simulink model "Wind_Turbine_test"  (R2023b)
settings: Solver=VariableStepAuto  StartTime=0.0  StopTime=1  RelTol=1e-3
model workspace (MAT data in the model file):
  Compensation_Ki = 30
  Compensation_Kp = 3
  DC_Ki = 400
  DC_Kp = 8
  F = 0.01
  Flux_min = 0.5
  Grid_Freq_PWM = 2700
  Grid_Ireg_Ki = 5
  Grid_Ireg_Kp = 0.83
  Grid_Ireg_lim = 1.1
  Grid_Modindex_Upper = 1.1
  Grid_conv_Imax = 0.8
  H = 0.685
  Idref_max = 0.9
  Iqref_Tc = 0.3
  Ki_Var = 0.05
  Ki_Vreg = 20
  Ksh = 1.1
  L_pu = 0.3
  Llr = 0.16
  Lls = 0.18
  Lm = 2.9
  P_mech = 1080000
  Pitch_Ki = 0
  Pitch_Kp = 150
  Pitch_Max = 27
  Pitch_Tc = 0.01
  Pitch_rate = 10
  Q_Filt = 50
  R_pu = 0.003
  Rotor_Freq_PWM = 1620
  Rotor_Ireg_Ki = 8
  Rotor_Ireg_Kp = 0.6
  Rotor_Ireg_lim = 0.1
  Rotor_Modindex_Upper = 2
  Rr = 0.016
  Rs = 0.023
  T_set = 0.0001
  Tp = 5e-05
  Ts = 5e-06
  Var_C_Filt = 720000
  Var_reg_max = 1.1
  Var_reg_min = 0.9
  WT_Coeff = [0.645 116 0.4 5 21 0.00912 0.08 0.035]
  WT_H = 4.32
  WT_IGBTRon = 5.931
  WT_Param = [91.204 10143]
  Wind_Freq_Filt = 10000
  Wind_Freq_nom = 60
  Wind_P_nom = 1200000
  Wind_Rotor_V_nom = 1950
  Wind_V_nom = 500
  Zeta_Filt = 0.707106781187
  init = [-0.2 0 0 0 0 0 0 0]
  p = 3
  torque0 = 0.83
  v_Ki = 0.1
  v_Kp = 3.6
  v_Max = 1.2
  v_Min = 0.7
  v_T = 5
  vreg_max = 1
  wind_VDC_nom = 1150
  wt0 = 1.2
undefined symbols (not defined in the file): D1, D11, Delta, DiscIntNeverNeededParam, P, Q
libraries: powerlib_extras x144, simulink_extras x24, spsThreePhaseVIMeasurementLib x13, spsThreePhaseTransformerTwoWindingsLib x11, spsSeriesRLCBranchLib x9, spsPWMGenerator2LevelLib x8, spsUniversalBridgeLib x8, spsThreePhaseSeriesRLCLoadLib x6, spsThreePhasePISectionLineLib x5, spsGroundLib x5, spsLoadFlowBusLib x4, spsAsynchronousMachinepuUnitsLib x4
(part 4 of 9)

== system Wind_Turbine_test/Wind Farm/Wind Turbine 1/Wind Turbine & Generator 1/Shaft ==
  Speed : Inport
  Discrete-Time Integrator1 : DiscreteIntegrator  InitialCondition=torque0/Ksh  SampleTime=Ts  ICPrevOutput=DiscIntNeverNeededParam  ICPrevScaledInput=DiscIntNeverNeededParam
  Mutual damping : Gain  Gain=1.5  SaturateOnIntegerOverflow=on  OutDataTypeStr=Inherit: Same as input  ParamDataTypeStr=Inherit: Same as input
  Stiffness : Gain  Gain=Ksh  SaturateOnIntegerOverflow=on  OutDataTypeStr=Inherit: Same as input  ParamDataTypeStr=Inherit: Same as input
  Sum2 : Sum  InputSameDT=on  SaturateOnIntegerOverflow=on  OutDataTypeStr=Inherit: Same as first input
  wbase : Gain  Gain=125.7  SaturateOnIntegerOverflow=on  OutDataTypeStr=Inherit: Same as input  ParamDataTypeStr=Inherit: Same as input
  T_shaft (pu) : Outport  VectorParamsAs1DForOutWhenUnconnected=off
  wires:
  Mutual damping/1 -> Sum2/2
  Stiffness/1 -> Sum2/1
  Sum2/1 -> T_shaft (pu)/1
  Speed/1 -> Mutual damping/1, wbase/1
  Discrete-Time Integrator1/1 -> Stiffness/1
  wbase/1 -> Discrete-Time Integrator1/1

== system Wind_Turbine_test/Wind Farm/Wind Turbine 1/Wind Turbine & Generator 1/Turbine ==
  T_wt (pu) : Inport
  T_shaft (pu) : Inport  Port=2
  Generator speed (pu) : Inport  Port=3
  1_2H_WT : Gain  Gain=1/(2*WT_H)  SaturateOnIntegerOverflow=on  OutDataTypeStr=Inherit: Same as input  ParamDataTypeStr=Inherit: Same as input
  Discrete-Time Integrator : DiscreteIntegrator  InitialCondition=wt0  SampleTime=Ts  ICPrevOutput=DiscIntNeverNeededParam  ICPrevScaledInput=DiscIntNeverNeededParam
  Sum : Sum  Inputs=+-  InputSameDT=on  SaturateOnIntegerOverflow=on  OutDataTypeStr=Inherit: Same as first input
  Sum1 : Sum  Inputs=+-  InputSameDT=on  SaturateOnIntegerOverflow=on  OutDataTypeStr=Inherit: Same as first input
  Turbine speed : Outport
  W_wt (pu) : Outport  Port=2  VectorParamsAs1DForOutWhenUnconnected=off
  wires:
  Sum1/1 -> Turbine speed/1
  Sum/1 -> 1_2H_WT/1
  Discrete-Time Integrator/1 -> W_wt (pu)/1, Sum1/1
  1_2H_WT/1 -> Discrete-Time Integrator/1
  T_wt (pu)/1 -> Sum/1
  T_shaft (pu)/1 -> Sum/2
  Generator speed (pu)/1 -> Sum1/2

== system Wind_Turbine_test/Wind Farm/Wind Turbine 1/Wind Turbine & Generator 1/Wind Turbine  ==
  Generator speed (pu)1 : Inport
  Pitch angle (deg) : Inport  Port=2
  Wind speed (m/s) : Inport  Port=3
  ->pu : Gain  Gain=1/Pmech_Out
  Avoid div. by zero : Saturate  UpperLimit=inf  LowerLimit=eps
  "Avoid div. by zero " : Saturate  UpperLimit=inf  LowerLimit=eps
  Fcn1 : Fcn  Expr=WT_Param(1)*u[2]/u[1]
  Fcn2 : Fcn  Expr=WT_Coeff8(1)*(WT_Coeff8(6)*u[1] + (-WT_Coeff8(4) - WT_Coeff8(3)*(2.5 + u[2]) + WT_Coeff8(2)*(1/(u[1] + WT_Coeff8(7)*(2.5 + u[2])) -WT_Coeff8(8)/(1 + (2.5 + u[2])^3)))/exp(WT_Coeff8(5)*(1/(u[1] + WT_Coeff8(7)*(2.5 + u[2])) - WT_Coeff8(8)/(1 + (2.5 + u[2])^3))))
  "K2*Cp*wind^3 " : Fcn  Expr=WT_Param(2)*u[1]^3*u[2]
  Mux : Mux  Inputs=2
  Mux1 : Mux  Inputs=2
  Mux2 : Mux  Inputs=2
  Product2 : Product  Inputs=*/  InputSameDT=on  SaturateOnIntegerOverflow=on  OutDataTypeStr=Inherit: Same as first input
  Tt (pu) : Outport  VectorParamsAs1DForOutWhenUnconnected=off
  wires:
  Generator speed (pu)1/1 -> "Avoid div. by zero "/1
  Mux1/1 -> Fcn2/1
  ->pu/1 -> Product2/1  "power_pu"
  Avoid div. by zero/1 -> Mux/1, Mux2/1
  "Avoid div. by zero "/1 -> Product2/2, Mux/2
  "K2*Cp*wind^3 "/1 -> ->pu/1
  Mux2/1 -> "K2*Cp*wind^3 "/1
  Fcn1/1 -> Mux1/1  "lambda"
  Mux/1 -> Fcn1/1
  Pitch angle (deg)/1 -> Mux1/2
  Wind speed (m/s)/1 -> Avoid div. by zero/1
  Product2/1 -> Tt (pu)/1
  Fcn2/1 -> Mux2/2  "Cp"

== system Wind_Turbine_test/Wind Farm/Wind Turbine 2/Wind Turbine & Generator 1/Shaft ==
  Speed : Inport
  Discrete-Time Integrator1 : DiscreteIntegrator  InitialCondition=torque0/Ksh  SampleTime=Ts  ICPrevOutput=DiscIntNeverNeededParam  ICPrevScaledInput=DiscIntNeverNeededParam
  Mutual damping : Gain  Gain=1.5  SaturateOnIntegerOverflow=on  OutDataTypeStr=Inherit: Same as input  ParamDataTypeStr=Inherit: Same as input
  Stiffness : Gain  Gain=Ksh  SaturateOnIntegerOverflow=on  OutDataTypeStr=Inherit: Same as input  ParamDataTypeStr=Inherit: Same as input
  Sum2 : Sum  InputSameDT=on  SaturateOnIntegerOverflow=on  OutDataTypeStr=Inherit: Same as first input
  wbase : Gain  Gain=125.7  SaturateOnIntegerOverflow=on  OutDataTypeStr=Inherit: Same as input  ParamDataTypeStr=Inherit: Same as input
  T_shaft (pu) : Outport  VectorParamsAs1DForOutWhenUnconnected=off
  wires:
  Mutual damping/1 -> Sum2/2
  Stiffness/1 -> Sum2/1
  Sum2/1 -> T_shaft (pu)/1
  Speed/1 -> Mutual damping/1, wbase/1
  Discrete-Time Integrator1/1 -> Stiffness/1
  wbase/1 -> Discrete-Time Integrator1/1

== system Wind_Turbine_test/Wind Farm/Wind Turbine 2/Wind Turbine & Generator 1/Turbine ==
  T_wt (pu) : Inport
  T_shaft (pu) : Inport  Port=2
  Generator speed (pu) : Inport  Port=3
  1_2H_WT : Gain  Gain=1/(2*WT_H)  SaturateOnIntegerOverflow=on  OutDataTypeStr=Inherit: Same as input  ParamDataTypeStr=Inherit: Same as input
  Discrete-Time Integrator : DiscreteIntegrator  InitialCondition=wt0  SampleTime=Ts  ICPrevOutput=DiscIntNeverNeededParam  ICPrevScaledInput=DiscIntNeverNeededParam
  Sum : Sum  Inputs=+-  InputSameDT=on  SaturateOnIntegerOverflow=on  OutDataTypeStr=Inherit: Same as first input
  Sum1 : Sum  Inputs=+-  InputSameDT=on  SaturateOnIntegerOverflow=on  OutDataTypeStr=Inherit: Same as first input
  Turbine speed : Outport
  W_wt (pu) : Outport  Port=2  VectorParamsAs1DForOutWhenUnconnected=off
  wires:
  Sum1/1 -> Turbine speed/1
  Sum/1 -> 1_2H_WT/1
  Discrete-Time Integrator/1 -> W_wt (pu)/1, Sum1/1
  1_2H_WT/1 -> Discrete-Time Integrator/1
  T_wt (pu)/1 -> Sum/1
  T_shaft (pu)/1 -> Sum/2
  Generator speed (pu)/1 -> Sum1/2

== system Wind_Turbine_test/Wind Farm/Wind Turbine 2/Wind Turbine & Generator 1/Wind Turbine  ==
  Generator speed (pu)1 : Inport
  Pitch angle (deg) : Inport  Port=2
  Wind speed (m/s) : Inport  Port=3
  ->pu : Gain  Gain=1/Pmech_Out
  Avoid div. by zero : Saturate  UpperLimit=inf  LowerLimit=eps
  "Avoid div. by zero " : Saturate  UpperLimit=inf  LowerLimit=eps
  Fcn1 : Fcn  Expr=WT_Param(1)*u[2]/u[1]
  Fcn2 : Fcn  Expr=WT_Coeff8(1)*(WT_Coeff8(6)*u[1] + (-WT_Coeff8(4) - WT_Coeff8(3)*(2.5 + u[2]) + WT_Coeff8(2)*(1/(u[1] + WT_Coeff8(7)*(2.5 + u[2])) -WT_Coeff8(8)/(1 + (2.5 + u[2])^3)))/exp(WT_Coeff8(5)*(1/(u[1] + WT_Coeff8(7)*(2.5 + u[2])) - WT_Coeff8(8)/(1 + (2.5 + u[2])^3))))
  "K2*Cp*wind^3 " : Fcn  Expr=WT_Param(2)*u[1]^3*u[2]
  Mux : Mux  Inputs=2
  Mux1 : Mux  Inputs=2
  Mux2 : Mux  Inputs=2
  Product2 : Product  Inputs=*/  InputSameDT=on  SaturateOnIntegerOverflow=on  OutDataTypeStr=Inherit: Same as first input
  Tt (pu) : Outport  VectorParamsAs1DForOutWhenUnconnected=off
  wires:
  Generator speed (pu)1/1 -> "Avoid div. by zero "/1
  Mux1/1 -> Fcn2/1
  ->pu/1 -> Product2/1  "power_pu"
  Avoid div. by zero/1 -> Mux/1, Mux2/1
  "Avoid div. by zero "/1 -> Product2/2, Mux/2
  "K2*Cp*wind^3 "/1 -> ->pu/1
  Mux2/1 -> "K2*Cp*wind^3 "/1
  Fcn1/1 -> Mux1/1  "lambda"
  Mux/1 -> Fcn1/1
  Pitch angle (deg)/1 -> Mux1/2
  Wind speed (m/s)/1 -> Avoid div. by zero/1
  Product2/1 -> Tt (pu)/1
  Fcn2/1 -> Mux2/2  "Cp"

== system Wind_Turbine_test/Wind Farm/Wind Turbine 3/Wind Turbine & Generator 1/Shaft ==
  Speed : Inport
  Discrete-Time Integrator1 : DiscreteIntegrator  InitialCondition=torque0/Ksh  SampleTime=Ts  ICPrevOutput=DiscIntNeverNeededParam  ICPrevScaledInput=DiscIntNeverNeededParam
  Mutual damping : Gain  Gain=1.5  SaturateOnIntegerOverflow=on  OutDataTypeStr=Inherit: Same as input  ParamDataTypeStr=Inherit: Same as input
  Stiffness : Gain  Gain=Ksh  SaturateOnIntegerOverflow=on  OutDataTypeStr=Inherit: Same as input  ParamDataTypeStr=Inherit: Same as input
  Sum2 : Sum  InputSameDT=on  SaturateOnIntegerOverflow=on  OutDataTypeStr=Inherit: Same as first input
  wbase : Gain  Gain=125.7  SaturateOnIntegerOverflow=on  OutDataTypeStr=Inherit: Same as input  ParamDataTypeStr=Inherit: Same as input
  T_shaft (pu) : Outport  VectorParamsAs1DForOutWhenUnconnected=off
  wires:
  Mutual damping/1 -> Sum2/2
  Stiffness/1 -> Sum2/1
  Sum2/1 -> T_shaft (pu)/1
  Speed/1 -> Mutual damping/1, wbase/1
  Discrete-Time Integrator1/1 -> Stiffness/1
  wbase/1 -> Discrete-Time Integrator1/1

== system Wind_Turbine_test/Wind Farm/Wind Turbine 3/Wind Turbine & Generator 1/Turbine ==
  T_wt (pu) : Inport
  T_shaft (pu) : Inport  Port=2
  Generator speed (pu) : Inport  Port=3
  1_2H_WT : Gain  Gain=1/(2*WT_H)  SaturateOnIntegerOverflow=on  OutDataTypeStr=Inherit: Same as input  ParamDataTypeStr=Inherit: Same as input
  Discrete-Time Integrator : DiscreteIntegrator  InitialCondition=wt0  SampleTime=Ts  ICPrevOutput=DiscIntNeverNeededParam  ICPrevScaledInput=DiscIntNeverNeededParam
  Sum : Sum  Inputs=+-  InputSameDT=on  SaturateOnIntegerOverflow=on  OutDataTypeStr=Inherit: Same as first input
  Sum1 : Sum  Inputs=+-  InputSameDT=on  SaturateOnIntegerOverflow=on  OutDataTypeStr=Inherit: Same as first input
  Turbine speed : Outport
  W_wt (pu) : Outport  Port=2  VectorParamsAs1DForOutWhenUnconnected=off
  wires:
  Sum1/1 -> Turbine speed/1
  Sum/1 -> 1_2H_WT/1
  Discrete-Time Integrator/1 -> W_wt (pu)/1, Sum1/1
  1_2H_WT/1 -> Discrete-Time Integrator/1
  T_wt (pu)/1 -> Sum/1
  T_shaft (pu)/1 -> Sum/2
  Generator speed (pu)/1 -> Sum1/2

== system Wind_Turbine_test/Wind Farm/Wind Turbine 3/Wind Turbine & Generator 1/Wind Turbine  ==
  Generator speed (pu)1 : Inport
  Pitch angle (deg) : Inport  Port=2
  Wind speed (m/s) : Inport  Port=3
  ->pu : Gain  Gain=1/Pmech_Out
  Avoid div. by zero : Saturate  UpperLimit=inf  LowerLimit=eps
  "Avoid div. by zero " : Saturate  UpperLimit=inf  LowerLimit=eps
  Fcn1 : Fcn  Expr=WT_Param(1)*u[2]/u[1]
  Fcn2 : Fcn  Expr=WT_Coeff8(1)*(WT_Coeff8(6)*u[1] + (-WT_Coeff8(4) - WT_Coeff8(3)*(2.5 + u[2]) + WT_Coeff8(2)*(1/(u[1] + WT_Coeff8(7)*(2.5 + u[2])) -WT_Coeff8(8)/(1 + (2.5 + u[2])^3)))/exp(WT_Coeff8(5)*(1/(u[1] + WT_Coeff8(7)*(2.5 + u[2])) - WT_Coeff8(8)/(1 + (2.5 + u[2])^3))))
  "K2*Cp*wind^3 " : Fcn  Expr=WT_Param(2)*u[1]^3*u[2]
  Mux : Mux  Inputs=2
  Mux1 : Mux  Inputs=2
  Mux2 : Mux  Inputs=2
  Product2 : Product  Inputs=*/  InputSameDT=on  SaturateOnIntegerOverflow=on  OutDataTypeStr=Inherit: Same as first input
  Tt (pu) : Outport  VectorParamsAs1DForOutWhenUnconnected=off
  wires:
  Generator speed (pu)1/1 -> "Avoid div. by zero "/1
  Mux1/1 -> Fcn2/1
  ->pu/1 -> Product2/1  "power_pu"
  Avoid div. by zero/1 -> Mux/1, Mux2/1
  "Avoid div. by zero "/1 -> Product2/2, Mux/2
  "K2*Cp*wind^3 "/1 -> ->pu/1
  Mux2/1 -> "K2*Cp*wind^3 "/1
  Fcn1/1 -> Mux1/1  "lambda"
  Mux/1 -> Fcn1/1
  Pitch angle (deg)/1 -> Mux1/2
  Wind speed (m/s)/1 -> Avoid div. by zero/1
  Product2/1 -> Tt (pu)/1
  Fcn2/1 -> Mux2/2  "Cp"

== system Wind_Turbine_test/Wind Farm/Wind Turbine 4/Wind Turbine & Generator 1/Shaft ==
  Speed : Inport
  Discrete-Time Integrator1 : DiscreteIntegrator  InitialCondition=torque0/Ksh  SampleTime=Ts  ICPrevOutput=DiscIntNeverNeededParam  ICPrevScaledInput=DiscIntNeverNeededParam
  Mutual damping : Gain  Gain=1.5  SaturateOnIntegerOverflow=on  OutDataTypeStr=Inherit: Same as input  ParamDataTypeStr=Inherit: Same as input
  Stiffness : Gain  Gain=Ksh  SaturateOnIntegerOverflow=on  OutDataTypeStr=Inherit: Same as input  ParamDataTypeStr=Inherit: Same as input
  Sum2 : Sum  InputSameDT=on  SaturateOnIntegerOverflow=on  OutDataTypeStr=Inherit: Same as first input
  wbase : Gain  Gain=125.7  SaturateOnIntegerOverflow=on  OutDataTypeStr=Inherit: Same as input  ParamDataTypeStr=Inherit: Same as input
  T_shaft (pu) : Outport  VectorParamsAs1DForOutWhenUnconnected=off
  wires:
  Mutual damping/1 -> Sum2/2
  Stiffness/1 -> Sum2/1
  Sum2/1 -> T_shaft (pu)/1
  Speed/1 -> Mutual damping/1, wbase/1
  Discrete-Time Integrator1/1 -> Stiffness/1
  wbase/1 -> Discrete-Time Integrator1/1

== system Wind_Turbine_test/Wind Farm/Wind Turbine 4/Wind Turbine & Generator 1/Turbine ==
  T_wt (pu) : Inport
  T_shaft (pu) : Inport  Port=2
  Generator speed (pu) : Inport  Port=3
  1_2H_WT : Gain  Gain=1/(2*WT_H)  SaturateOnIntegerOverflow=on  OutDataTypeStr=Inherit: Same as input  ParamDataTypeStr=Inherit: Same as input
  Discrete-Time Integrator : DiscreteIntegrator  InitialCondition=wt0  SampleTime=Ts  ICPrevOutput=DiscIntNeverNeededParam  ICPrevScaledInput=DiscIntNeverNeededParam
  Sum : Sum  Inputs=+-  InputSameDT=on  SaturateOnIntegerOverflow=on  OutDataTypeStr=Inherit: Same as first input
  Sum1 : Sum  Inputs=+-  InputSameDT=on  SaturateOnIntegerOverflow=on  OutDataTypeStr=Inherit: Same as first input
  Turbine speed : Outport
  W_wt (pu) : Outport  Port=2  VectorParamsAs1DForOutWhenUnconnected=off
  wires:
  Sum1/1 -> Turbine speed/1
  Sum/1 -> 1_2H_WT/1
  Discrete-Time Integrator/1 -> W_wt (pu)/1, Sum1/1
  1_2H_WT/1 -> Discrete-Time Integrator/1
  T_wt (pu)/1 -> Sum/1
  T_shaft (pu)/1 -> Sum/2
  Generator speed (pu)/1 -> Sum1/2

== system Wind_Turbine_test/Wind Farm/Wind Turbine 4/Wind Turbine & Generator 1/Wind Turbine  ==
  Generator speed (pu)1 : Inport
  Pitch angle (deg) : Inport  Port=2
  Wind speed (m/s) : Inport  Port=3
  ->pu : Gain  Gain=1/Pmech_Out
  Avoid div. by zero : Saturate  UpperLimit=inf  LowerLimit=eps
  "Avoid div. by zero " : Saturate  UpperLimit=inf  LowerLimit=eps
  Fcn1 : Fcn  Expr=WT_Param(1)*u[2]/u[1]
  Fcn2 : Fcn  Expr=WT_Coeff8(1)*(WT_Coeff8(6)*u[1] + (-WT_Coeff8(4) - WT_Coeff8(3)*(2.5 + u[2]) + WT_Coeff8(2)*(1/(u[1] + WT_Coeff8(7)*(2.5 + u[2])) -WT_Coeff8(8)/(1 + (2.5 + u[2])^3)))/exp(WT_Coeff8(5)*(1/(u[1] + WT_Coeff8(7)*(2.5 + u[2])) - WT_Coeff8(8)/(1 + (2.5 + u[2])^3))))
  "K2*Cp*wind^3 " : Fcn  Expr=WT_Param(2)*u[1]^3*u[2]
  Mux : Mux  Inputs=2
  Mux1 : Mux  Inputs=2
  Mux2 : Mux  Inputs=2
  Product2 : Product  Inputs=*/  InputSameDT=on  SaturateOnIntegerOverflow=on  OutDataTypeStr=Inherit: Same as first input
  Tt (pu) : Outport  VectorParamsAs1DForOutWhenUnconnected=off
  wires:
  Generator speed (pu)1/1 -> "Avoid div. by zero "/1
  Mux1/1 -> Fcn2/1
  ->pu/1 -> Product2/1  "power_pu"
  Avoid div. by zero/1 -> Mux/1, Mux2/1
  "Avoid div. by zero "/1 -> Product2/2, Mux/2
  "K2*Cp*wind^3 "/1 -> ->pu/1
  Mux2/1 -> "K2*Cp*wind^3 "/1
  Fcn1/1 -> Mux1/1  "lambda"
  Mux/1 -> Fcn1/1
  Pitch angle (deg)/1 -> Mux1/2
  Wind speed (m/s)/1 -> Avoid div. by zero/1
  Product2/1 -> Tt (pu)/1
  Fcn2/1 -> Mux2/2  "Cp"

== system Wind_Turbine_test/Wind Farm/Control System/Control System 1/Grid-side Control System/Current Regulator ==
  Stator_Vdq : Inport
  In2 : Inport  Port=2
  Grid_conv_Idq : Inport  Port=3
  w : Inport  Port=4
  Constant1 : Constant  Value=L_pu
  Constant2 : Constant  Value=L_pu
  Constant3 : Constant  Value=R_pu
  Constant4 : Constant  Value=R_pu
  Demux{,1..3} (4 alike) : Demux  Outputs=2
      settings: DisplayOption=none
  Discrete PI Controller1 : powerlib_extras/Discrete  Control Blocks/Discrete PI Controller  Kp=Grid_Ireg_Kp  Ki=Grid_Ireg_Ki  Par_Limits=[1.0 -1.0] *Grid_Ireg_lim  Init=0  Ts=Ts
  Mux2 : Mux  Inputs=2
  Product : Product  Inputs=3  InputSameDT=on  SaturateOnIntegerOverflow=on  OutDataTypeStr=Inherit: Same as first input
  Product1 : Product  Inputs=3  InputSameDT=on  SaturateOnIntegerOverflow=on  OutDataTypeStr=Inherit: Same as first input
  Product2 : Product  InputSameDT=on  SaturateOnIntegerOverflow=on  OutDataTypeStr=Inherit: Same as first input
  Product3 : Product  InputSameDT=on  SaturateOnIntegerOverflow=on  OutDataTypeStr=Inherit: Same as first input
  Sum1 : Sum  Inputs=+-  InputSameDT=on  SaturateOnIntegerOverflow=on  OutDataTypeStr=Inherit: Same as first input
  Sum2 : Sum  Inputs=-+|  InputSameDT=on  SaturateOnIntegerOverflow=on  OutDataTypeStr=Inherit: Same as first input
  Sum3 : Sum  Inputs=||++-  InputSameDT=on  SaturateOnIntegerOverflow=on  OutDataTypeStr=Inherit: Same as first input
  Sum4 : Sum  Inputs=|+-  InputSameDT=on  SaturateOnIntegerOverflow=on  OutDataTypeStr=Inherit: Same as first input
  Sum5 : Sum  Inputs=|--+  InputSameDT=on  SaturateOnIntegerOverflow=on  OutDataTypeStr=Inherit: Same as first input
  Sum6 : Sum  Inputs=|-+  InputSameDT=on  SaturateOnIntegerOverflow=on  OutDataTypeStr=Inherit: Same as first input
  Grid_conv_Vd : Outport
  Grid_conv_Vq : Outport  Port=2
  wires:
  Product1/1 -> Sum5/2
  Product2/1 -> Sum3/3
  Product3/1 -> Sum5/1
  [id_ref] -> Product2/2
  Sum1/1 -> Grid_conv_Vd/1  "Grid_conv_Vd"
  Demux1/2 -> [iq_ref], Sum2/2  "Iq_ref"
  Demux/1 -> Sum4/2  "Id"
  [w] -> Product/2
  Demux2/2 -> Sum5/3  "Vq"
  [iq_ref] -> Product/3
  Sum4/1 -> Mux2/1
  Constant4/1 -> Product3/2
  Stator_Vdq/1 -> Demux2/1
  Constant2/1 -> Product1/2
  Constant3/1 -> Product2/1
  Grid_conv_Idq/1 -> Demux/1
  Product/1 -> Sum3/2
  Discrete PI Controller1/1 -> Demux3/1
  Sum2/1 -> Mux2/2
  Sum6/1 -> Grid_conv_Vq/1  "Grid_conv_Vq"
  w/1 -> [w]
  [id_ref] -> Product1/1
  Sum5/1 -> Sum6/2
  [iq_ref] -> Product3/1
  Sum3/1 -> Sum1/1
  Mux2/1 -> Discrete PI Controller1/1
  Demux2/1 -> Sum3/1  "Vd"
  Demux1/1 -> Sum4/1, [id_ref]  "Id_ref"
  Demux3/1 -> Sum1/2  "vd'"
  Constant1/1 -> Product/1
  Demux/2 -> Sum2/1  "Iq"
  Demux3/2 -> Sum6/1  "vq'"
  [w] -> Product1/3
  In2/1 -> Demux1/1

== system Wind_Turbine_test/Wind Farm/Control System/Control System 1/Grid-side Control System/Grid Voltage Converter ==
  dq0 : Inport
  Theta_PLL : Inport  Port=2
  Mux5 : Mux  Inputs=2
  Trigonometric Function2 : Trigonometry
  Trigonometric Function3 : Trigonometry  Operator=cos
  dq0_to_abc Transformation : powerlib_extras/Measurements/dq0_to_abc Transformation
  Grid_conv_V : Outport  VectorParamsAs1DForOutWhenUnconnected=off
  wires:
  Trigonometric Function2/1 -> Mux5/1
  Mux5/1 -> dq0_to_abc Transformation/2
  Theta_PLL/1 -> Trigonometric Function2/1, Trigonometric Function3/1
  dq0_to_abc Transformation/1 -> Grid_conv_V/1
  dq0/1 -> dq0_to_abc Transformation/1
  Trigonometric Function3/1 -> Mux5/2

== system Wind_Turbine_test/Wind Farm/Control System/Control System 1/Grid-side Control System/Modulation ==
  x : Inport
  y : Inport  Port=2
  1 : Saturate  UpperLimit=Grid_Modindex_Upper  LowerLimit=0
  Avoid division by zero : Saturate  UpperLimit=inf  LowerLimit=1e-6
  Cartesian to Polar1 : simulink_extras/Transformations/Cartesian to Polar
  K : Constant  Value=Wind_V_nom*2*sqrt(2/3)
  Mux4 : Mux  Inputs=3
  Polar to Cartesian : simulink_extras/Transformations/Polar to Cartesian
  Product4 : Product  Inputs=**/  InputSameDT=on  SaturateOnIntegerOverflow=on  OutDataTypeStr=Inherit: Same as first input
  V0 : Constant  Value=0
  Vdq0 : Outport
  wires:
  K/1 -> Product4/2
  Polar to Cartesian/2 -> Mux4/2
  V0/1 -> Mux4/3
  y/1 -> Cartesian to Polar1/2
  [Vdc] -> Avoid division by zero/1
  Polar to Cartesian/1 -> Mux4/1
  Mux4/1 -> Vdq0/1  "Vdq0"
  Avoid division by zero/1 -> Product4/3
  1/1 -> Polar to Cartesian/1
  Cartesian to Polar1/2 -> Polar to Cartesian/2
  Product4/1 -> 1/1  "m"
  x/1 -> Cartesian to Polar1/1
  Cartesian to Polar1/1 -> Product4/1

== system Wind_Turbine_test/Wind Farm/Control System/Control System 1/Grid-side Control System/VDC Regulator ==
  Iq_ref : Inport
  Vdc : Inport  Port=2
  ->pu : Gain  Gain=1/wind_VDC_nom
  Discrete PI Controller : powerlib_extras/Discrete  Control Blocks/Discrete PI Controller  Kp=DC_Kp  Ki=DC_Ki  Par_Limits=[1 -1]*Grid_conv_Imax  Init=0  Ts=Ts
  Mux : Mux  Inputs=2
  Sum7 : Sum  Inputs=|+-  InputSameDT=on  SaturateOnIntegerOverflow=on  OutDataTypeStr=Inherit: Same as first input
  Vdc_ref (V) : Constant  Value=wind_VDC_nom
  Out1 : Outport
  wires:
  Vdc/1 -> [Vdc], Sum7/2
  Iq_ref/1 -> Mux/2
  Mux/1 -> Out1/1
  Discrete PI Controller/1 -> Mux/1  "Id_ref"
  ->pu/1 -> Discrete PI Controller/1
  Vdc_ref (V)/1 -> Sum7/1
  Sum7/1 -> ->pu/1

== system Wind_Turbine_test/Wind Farm/Control System/Control System 1/Measurement and abc-to-dq transformation / Improved Discrete 3-phase PLL ==
  note: Pierre Giroux, Gilbert Sybille, R. Gagnon
      | Power System Laboratory, IREQ
      | Hydro-Quebec
  note: New Discrete 3-phase PLL
  Vabc_pu : Inport  PortDimensions=3
  2nd-Order Filter : powerlib_extras/Discrete  Control Blocks/Discrete  2nd-Order Filter  FilterType=Lowpass  Fo=25  Zeta=0.707  Ts=Ts  Initialize=on  Vac_Init=[0 0 Finit]  Vdc_Init=Finit  PlotResponse=off  param1=[1 500 0.1]
  Constant1 : Constant  Value=2*pi*Finit
  Constant4 : Constant  Value=2*pi
  Discrete-Time Integrator : DiscreteIntegrator  SampleTime=Ts  ICPrevOutput=DiscIntNeverNeededParam  ICPrevScaledInput=DiscIntNeverNeededParam
  Discrete-Time Integrator1 : DiscreteIntegrator  gainval=1  SampleTime=Ts  LimitOutput=on  UpperSaturationLimit=2*pi*5  LowerSaturationLimit=-2*pi*5  ICPrevOutput=DiscIntNeverNeededParam  ICPrevScaledInput=DiscIntNeverNeededParam
  Gain10 : Gain  Gain=1/2/pi  SaturateOnIntegerOverflow=on  OutDataTypeStr=Inherit: Same as input  ParamDataTypeStr=Inherit: Same as input
  Kp1 : Gain  Gain=Kp2  SaturateOnIntegerOverflow=on  OutDataTypeStr=Inherit: Same as input  ParamDataTypeStr=Inherit: Same as input
  Kp2 : Gain  Gain=Ki2  SaturateOnIntegerOverflow=on  OutDataTypeStr=Inherit: Same as input  ParamDataTypeStr=Inherit: Same as input
  Kp3 : Gain  Gain=Ki1  SaturateOnIntegerOverflow=on  OutDataTypeStr=Inherit: Same as input  ParamDataTypeStr=Inherit: Same as input
  Kp4 : Gain  Gain=Kp1  SaturateOnIntegerOverflow=on  OutDataTypeStr=Inherit: Same as input  ParamDataTypeStr=Inherit: Same as input
  Math Function : Math  Operator=mod  SignedPower=on
  Mux2 : Mux  Inputs=2
  Rate Limiter : powerlib_extras/Discrete  Control Blocks/Discrete Rate Limiter  R=12  F=-12  Vinit=Finit  Ts=Ts
  Selector : Selector  InputPortWidth=3  IndexOptions=Index vector (dialog)  Indices=2  OutputSizes=1
  Sum : Sum  Inputs=+++
  Trigonometric Function : Trigonometry
  Trigonometric Function1 : Trigonometry  Operator=atan
  Trigonometric Function2 : Trigonometry  Operator=cos
  Trigonometric Function3 : Trigonometry  Operator=atan
  Unit Delay : UnitDelay  InitialCondition=Finit  SampleTime=Ts  HasFrameUpgradeWarning=on
  Variable Frequency Mean value : powerlib_extras/Discrete Measurements/Discrete Variable Frequency Mean value  Finit=Finit  Fmin=Fmin  Vinit=0  Ts=Ts
  abc_to_dq0 Transformation : powerlib_extras/Measurements/abc_to_dq0 Transformation
  wind_Freq : Outport  VectorParamsAs1DForOutWhenUnconnected=off
  theta : Outport  Port=2  VectorParamsAs1DForOutWhenUnconnected=off
  Sin_Cos : Outport  Port=3  VectorParamsAs1DForOutWhenUnconnected=off
  wires:
  Discrete-Time Integrator1/1 -> Sum/2
  Kp1/1 -> Sum/1
  Discrete-Time Integrator/1 -> Math Function/1
  Unit Delay/1 -> Variable Frequency Mean value/1, wind_Freq/1
  Sum/1 -> Gain10/1, Discrete-Time Integrator/1
  Kp2/1 -> Discrete-Time Integrator1/1
  Trigonometric Function3/1 -> Kp2/1
  Kp3/1 -> Trigonometric Function3/1
  Variable Frequency Mean value/1 -> Kp3/1, Kp4/1
  Constant1/1 -> Sum/3
  Trigonometric Function1/1 -> Kp1/1
  Kp4/1 -> Trigonometric Function1/1
  Selector/1 -> Variable Frequency Mean value/2  "Vq"
  2nd-Order Filter/1 -> Unit Delay/1
  Rate Limiter/1 -> 2nd-Order Filter/1
  Gain10/1 -> Rate Limiter/1
  Mux2/1 -> abc_to_dq0 Transformation/2, Sin_Cos/1
  Trigonometric Function2/1 -> Mux2/2
  Trigonometric Function/1 -> Mux2/1
  Math Function/1 -> theta/1, Trigonometric Function2/1, Trigonometric Function/1
  Constant4/1 -> Math Function/2
  abc_to_dq0 Transformation/1 -> Selector/1
  Vabc_pu/1 -> abc_to_dq0 Transformation/1

== system Wind_Turbine_test/Wind Farm/Control System/Control System 1/Measurement and abc-to-dq transformation /Discrete 3-phase PLL-Driven Positive-Sequence  ==
  note: Discrete 3-phase PLL-driven Positive-Sequence Active & Reactive Power
  note: Pierre Giroux, Gilbert Sybille
      | Power System Simulation Laboratory
      | IREQ, Hydro-Quebc
  wind_Freq : Inport  PortDimensions=1
  Sin_Cos : Inport  Port=2  PortDimensions=2
  Vabc_V : Inport  Port=3  PortDimensions=3
  Iabc_A : Inport  Port=4  PortDimensions=3
  Deg->Rad : Gain  Gain=pi/180  SaturateOnIntegerOverflow=on  OutDataTypeStr=Inherit: Same as input  ParamDataTypeStr=Inherit: Same as input
  Discrete 3-phase PLL-Driven Positive-Sequence Fundamental Value : Subsystem  mask(Discrete 3-phase PLL-Driven Positive-Sequence Fundamental Value){Finit=Finit, Fmin=Fmin, Par_Init=Par_Vinit, Ts=Ts}
      mask prompts: Finit "Initial frequency (Hz):"; Fmin "Minimum frequency (Hz):"; Par_Init "Initial input (positive component): [ Mag  Phase-relative-to-PLL(degrees) ]"; Ts "Sample time:"
      mask help:
      | For a supplied fundamental frequency (port Freq), this discrete block computes  the positive-sequence component (Magnitude and Phase)  of a set of three balanced or unbalanced signals (port abc) which may contain harmonics.
      |  Input port "Sin_Cos" (a two-dimension signal) provides the reference frame required for the computation..
      |  First and second outputs return respectively the magnitude and phase (in degrees relative to the PLL phase)) of the fundamental.
      | For the first cycle of simulation, the outputs are held constant to the values specified by the parameter "Initial input".
      | constant to the values specified by the parameter "Initial input". The value of the parameter "Minimum frequency" is used to determine the buffer size of the "Variable Transport Delay" block found inside this subsystem.
      mask init:
      | Real_Init=Par_Init(1)*cos(pi/180*Par_Init(2));
      | Imag_Init=Par_Init(1)*sin(pi/180*Par_Init(2));
      | power_initmask();
      settings: OpenFcn=power_openblockproxy();
  Discrete 3-phase PLL-Driven Positive-Sequence Fundamental Value2 : Subsystem  mask(Discrete 3-phase PLL-Driven Positive-Sequence Fundamental Value){Finit=Finit, Fmin=Fmin, Par_Init=Par_Iinit, Ts=Ts}
      mask prompts: Finit "Initial frequency (Hz):"; Fmin "Minimum frequency (Hz):"; Par_Init "Initial input (positive component): [ Mag  Phase-relative-to-PLL(degrees) ]"; Ts "Sample time:"
      mask help:
      | For a supplied fundamental frequency (port Freq), this discrete block computes  the positive-sequence component (Magnitude and Phase)  of a set of three balanced or unbalanced signals (port abc) which may contain harmonics.
      |  Input port "Sin_Cos" (a two-dimension signal) provides the reference frame required for the computation..
      |  First and second outputs return respectively the magnitude and phase (in degrees relative to the PLL phase)) of the fundamental.
      | For the first cycle of simulation, the outputs are held constant to the values specified by the parameter "Initial input".
      | constant to the values specified by the parameter "Initial input". The value of the parameter "Minimum frequency" is used to determine the buffer size of the "Variable Transport Delay" block found inside this subsystem.
      mask init:
      | Real_Init=Par_Init(1)*cos(pi/180*Par_Init(2));
      | Imag_Init=Par_Init(1)*sin(pi/180*Par_Init(2));
      | power_initmask();
      settings: OpenFcn=power_openblockproxy();
  Gain1 : Gain  Gain=3/2  SaturateOnIntegerOverflow=on  OutDataTypeStr=Inherit: Same as input  ParamDataTypeStr=Inherit: Same as input
  Gain2 : Gain  Gain=3/2  SaturateOnIntegerOverflow=on  OutDataTypeStr=Inherit: Same as input  ParamDataTypeStr=Inherit: Same as input
  Product : Product  InputSameDT=on  SaturateOnIntegerOverflow=on  OutDataTypeStr=Inherit: Same as first input
  Product1 : Product  InputSameDT=on  SaturateOnIntegerOverflow=on  OutDataTypeStr=Inherit: Same as first input
  Product2 : Product  InputSameDT=on  SaturateOnIntegerOverflow=on  OutDataTypeStr=Inherit: Same as first input
  Sum : Sum  Inputs=+-  InputSameDT=on  SaturateOnIntegerOverflow=on  OutDataTypeStr=Inherit: Same as first input
  Trigonometric Function : Trigonometry
  Trigonometric Function1 : Trigonometry  Operator=cos
  Mag_V_V : Outport  VectorParamsAs1DForOutWhenUnconnected=off
  P_W : Outport  Port=2  VectorParamsAs1DForOutWhenUnconnected=off
  Q_Var : Outport  Port=3  VectorParamsAs1DForOutWhenUnconnected=off
  wires:
  Vabc_V/1 -> Discrete 3-phase PLL-Driven Positive-Sequence Fundamental Value/3(abc)
  wind_Freq/1 -> Discrete 3-phase PLL-Driven Positive-Sequence Fundamental Value/1(Freq), Discrete 3-phase PLL-Driven Positive-Sequence Fundamental Value2/1(Freq)
  Sin_Cos/1 -> Discrete 3-phase PLL-Driven Positive-Sequence Fundamental Value/2(Sin_Cos), Discrete 3-phase PLL-Driven Positive-Sequence Fundamental Value2/2(Sin_Cos)
  Discrete 3-phase PLL-Driven Positive-Sequence Fundamental Value/2(Phase) -> Sum/1
  Discrete 3-phase PLL-Driven Positive-Sequence Fundamental Value/1(Mag) -> Product2/1, Mag_V_V/1
  Discrete 3-phase PLL-Driven Positive-Sequence Fundamental Value2/2(Phase) -> Sum/2
  Sum/1 -> Deg->Rad/1
  Deg->Rad/1 -> Trigonometric Function1/1, Trigonometric Function/1
  Trigonometric Function1/1 -> Product/2
  Trigonometric Function/1 -> Product1/1
  Product/1 -> Gain1/1
  Gain1/1 -> P_W/1
  Product2/1 -> Product/1, Product1/2
  Discrete 3-phase PLL-Driven Positive-Sequence Fundamental Value2/1(Mag) -> Product2/2
  Iabc_A/1 -> Discrete 3-phase PLL-Driven Positive-Sequence Fundamental Value2/3(abc)
  Product1/1 -> Gain2/1
  Gain2/1 -> Q_Var/1

== system Wind_Turbine_test/Wind Farm/Control System/Control System 1/Measurement and abc-to-dq transformation /Filter ==
  Vabc : Inport
  Stator_Iabc : Inport  Port=2
  Iabc_grid_conv : Inport  Port=3
  Rotor_Iabc : Inport  Port=4
  Vdc : Inport  Port=5
  Qref : Inport  Port=6
  wr : Inport  Port=7
  angle_rotor : Inport  Port=8
  Demux{,1..3} (4 alike) : Demux  Outputs=3
      settings: DisplayOption=none
  Discrete 2nd-Order Filter{1..6,8..16} (15 alike) : powerlib_extras/Discrete  Control Blocks/Discrete  2nd-Order Filter  FilterType=Lowpass  Fo=Freq  Zeta=Zeta1  Ts=Ts  Initialize=off  Vac_Init=[0.8 -25 60]  Vdc_Init=-0.4  PlotResponse=off  param1=[1 500 1]
  Discrete 2nd-Order Filter7 : powerlib_extras/Discrete  Control Blocks/Discrete  2nd-Order Filter  FilterType=Lowpass  Fo=Freq  Zeta=Zeta1  Ts=Ts  Initialize=on  Vac_Init=[0.8 -25 60]*0  Vdc_Init=wind_VDC_nom  PlotResponse=off  param1=[1 500 1]
  Mux{,1..3} (4 alike) : Mux  Inputs=3
  "Vabc " : Outport  VectorParamsAs1DForOutWhenUnconnected=off
  "Stator_Iabc " : Outport  Port=2  VectorParamsAs1DForOutWhenUnconnected=off
  "Iabc_grid_conv " : Outport  Port=3  VectorParamsAs1DForOutWhenUnconnected=off
  "Rotor_Iabc " : Outport  Port=4  VectorParamsAs1DForOutWhenUnconnected=off
  "Vdc " : Outport  Port=5  VectorParamsAs1DForOutWhenUnconnected=off
  "Qref " : Outport  Port=6  VectorParamsAs1DForOutWhenUnconnected=off
  "wr " : Outport  Port=7  VectorParamsAs1DForOutWhenUnconnected=off
  "angle_rotor " : Outport  Port=8  VectorParamsAs1DForOutWhenUnconnected=off
  wires:
  Demux/1 -> Discrete 2nd-Order Filter1/1
  Demux/2 -> Discrete 2nd-Order Filter2/1
  Demux/3 -> Discrete 2nd-Order Filter3/1
  Discrete 2nd-Order Filter1/1 -> Mux/1
  Discrete 2nd-Order Filter2/1 -> Mux/2
  Discrete 2nd-Order Filter3/1 -> Mux/3
  Vabc/1 -> Demux/1
  Mux/1 -> "Vabc "/1
  Demux1/1 -> Discrete 2nd-Order Filter5/1
  Demux1/2 -> Discrete 2nd-Order Filter6/1
  Demux1/3 -> Discrete 2nd-Order Filter4/1
  Discrete 2nd-Order Filter5/1 -> Mux1/1
  Discrete 2nd-Order Filter6/1 -> Mux1/2
  Discrete 2nd-Order Filter4/1 -> Mux1/3
  Iabc_grid_conv/1 -> Demux1/1
  Mux1/1 -> "Iabc_grid_conv "/1
  Vdc/1 -> Discrete 2nd-Order Filter7/1
  Discrete 2nd-Order Filter7/1 -> "Vdc "/1
  Demux2/1 -> Discrete 2nd-Order Filter8/1
  Demux2/2 -> Discrete 2nd-Order Filter9/1
  Demux2/3 -> Discrete 2nd-Order Filter10/1
  Discrete 2nd-Order Filter8/1 -> Mux2/1
  Discrete 2nd-Order Filter9/1 -> Mux2/2
  Discrete 2nd-Order Filter10/1 -> Mux2/3
  Stator_Iabc/1 -> Demux2/1
  Mux2/1 -> "Stator_Iabc "/1
  wr/1 -> Discrete 2nd-Order Filter13/1
  Discrete 2nd-Order Filter13/1 -> "wr "/1
  Demux3/1 -> Discrete 2nd-Order Filter15/1
  Demux3/2 -> Discrete 2nd-Order Filter16/1
  Demux3/3 -> Discrete 2nd-Order Filter14/1
  Discrete 2nd-Order Filter15/1 -> Mux3/1
  Discrete 2nd-Order Filter16/1 -> Mux3/2
  Discrete 2nd-Order Filter14/1 -> Mux3/3
  Rotor_Iabc/1 -> Demux3/1
  Mux3/1 -> "Rotor_Iabc "/1
  Qref/1 -> Discrete 2nd-Order Filter11/1
  Discrete 2nd-Order Filter11/1 -> "Qref "/1
  angle_rotor/1 -> Discrete 2nd-Order Filter12/1
  Discrete 2nd-Order Filter12/1 -> "angle_rotor "/1

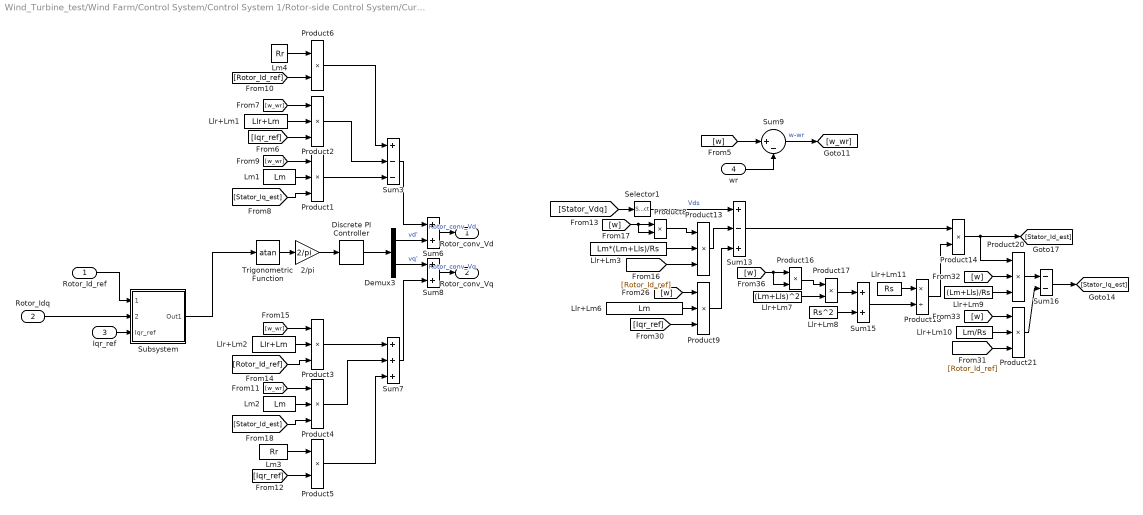
== system Wind_Turbine_test/Wind Farm/Control System/Control System 1/Rotor-side Control System/Current Regulator ==
  Rotor_Id_ref : Inport
  Rotor_Idq : Inport  Port=2
  Iqr_ref : Inport  Port=3
  wr : Inport  Port=4
  2/pi : Gain  Gain=2/pi
  Demux3 : Demux  Outputs=2
      settings: DisplayOption=none
  Discrete PI Controller : powerlib_extras/Discrete  Control Blocks/Discrete PI Controller  Kp=Rotor_Ireg_Kp  Ki=Rotor_Ireg_Ki  Par_Limits=[1 -1]* Rotor_Ireg_lim  Init=0  Ts=Ts
  Llr+Lm1 : Constant  Value=Llr+Lm
  Llr+Lm10 : Constant  Value=Lm/Rs
  Llr+Lm11 : Constant  Value=Rs
  Llr+Lm2 : Constant  Value=Llr+Lm
  Llr+Lm3 : Constant  Value=Lm*(Lm+Lls)/Rs
  Llr+Lm6 : Constant  Value=Lm
  Llr+Lm7 : Constant  Value=(Lm+Lls)^2
  Llr+Lm8 : Constant  Value=Rs^2
  Llr+Lm9 : Constant  Value=(Lm+Lls)/Rs
  Lm1 : Constant  Value=Lm
  Lm2 : Constant  Value=Lm
  Lm3 : Constant  Value=Rr
  Lm4 : Constant  Value=Rr  VectorParams1D=off
  Product{1..4,9,13,20..21} (8 alike) : Product  Inputs=3  SaturateOnIntegerOverflow=on  OutDataTypeStr=Inherit: Same as first input
  Product{5..6,8,14,16..17} (6 alike) : Product  SaturateOnIntegerOverflow=on  OutDataTypeStr=Inherit: Same as first input
  Product18 : Product  Inputs=*/  SaturateOnIntegerOverflow=on  OutDataTypeStr=Inherit: Same as first input
  Selector1 : Selector  InputPortWidth=2  IndexOptions=Index vector (dialog)  Indices=1  OutputSizes=[(-2)]
  Subsystem : Subsystem
  Sum13 : Sum  Inputs=+-+  InputSameDT=on  SaturateOnIntegerOverflow=on  OutDataTypeStr=Inherit: Same as first input
  Sum15 : Sum  InputSameDT=on  SaturateOnIntegerOverflow=on  OutDataTypeStr=Inherit: Same as first input
  Sum16 : Sum  Inputs=--  InputSameDT=on  SaturateOnIntegerOverflow=on  OutDataTypeStr=Inherit: Same as first input
  Sum3 : Sum  Inputs=+--  InputSameDT=on  SaturateOnIntegerOverflow=on  OutDataTypeStr=Inherit: Same as first input
  Sum6 : Sum  InputSameDT=on  SaturateOnIntegerOverflow=on  OutDataTypeStr=Inherit: Same as first input
  Sum7 : Sum  Inputs=+++  InputSameDT=on  SaturateOnIntegerOverflow=on  OutDataTypeStr=Inherit: Same as first input
  Sum8 : Sum  InputSameDT=on  SaturateOnIntegerOverflow=on  OutDataTypeStr=Inherit: Same as first input
  Sum9 : Sum  Inputs=|+-  InputSameDT=on  SaturateOnIntegerOverflow=on  OutDataTypeStr=Inherit: Same as first input
  Trigonometric Function : Trigonometry  Operator=atan
  Rotor_conv_Vd : Outport
  Rotor_conv_Vq : Outport  Port=2
  wires:
  Lm3/1 -> Product5/1
  Lm1/1 -> Product1/2
  Product8/1 -> Product13/1
  Sum8/1 -> Rotor_conv_Vq/1  "Rotor_conv_Vq"
  Selector1/1 -> Sum13/1  "Vds"
  Subsystem/1(Out1) -> Trigonometric Function/1
  Lm4/1 -> Product6/1
  Product13/1 -> Sum13/2
  Product6/1 -> Sum3/1
  Product1/1 -> Sum3/3
  Llr+Lm9/1 -> Product20/3
  Rotor_Idq/1 -> Subsystem/2(Rotor_Idq)
  Llr+Lm2/1 -> Product3/2
  Iqr_ref/1 -> Subsystem/3(Iqr_ref)
  [w_wr] -> Product4/1
  Product18/1 -> Product14/2
  [w] -> Product20/2
  Sum3/1 -> Sum6/1
  Sum15/1 -> Product18/2
  Sum7/1 -> Sum8/2
  [w] -> Product16/2, Product16/1
  [Rotor_Id_ref] -> Product6/2
  [w_wr] -> Product1/1
  Llr+Lm3/1 -> Product13/2
  Product21/1 -> Sum16/2
  [Iqr_ref] -> Product9/3
  [w_wr] -> Product3/1
  Product4/1 -> Sum7/2
  Product17/1 -> Sum15/1
  Llr+Lm11/1 -> Product18/1
  Demux3/2 -> Sum8/1  "vq'"
  [Stator_Id_est] -> Product4/3
  Product14/1 -> [Stator_Id_est], Product20/1
  [Rotor_Id_ref] -> Product21/3
  [Stator_Vdq] -> Selector1/1
  Sum16/1 -> [Stator_Iq_est]
  Llr+Lm8/1 -> Sum15/2
  Demux3/1 -> Sum6/2  "vd'"
  Lm2/1 -> Product4/2
  Product20/1 -> Sum16/1
  [w_wr] -> Product2/1
  [w] -> Product9/1
  Llr+Lm7/1 -> Product17/2
  [Iqr_ref] -> Product5/2
  Trigonometric Function/1 -> 2/pi/1
  Sum13/1 -> Product14/1
  [Rotor_Id_ref] -> Product3/3
  Llr+Lm1/1 -> Product2/2
  [Rotor_Id_ref] -> Product13/3
  Product5/1 -> Sum7/3
  [w] -> Sum9/1
  Sum9/1 -> [w_wr]  "w-wr"
  Discrete PI Controller/1 -> Demux3/1
  wr/1 -> Sum9/2
  Product9/1 -> Sum13/3
  [w] -> Product8/1, Product8/2
  Llr+Lm10/1 -> Product21/2
  2/pi/1 -> Discrete PI Controller/1
  [Stator_Iq_est] -> Product1/3
  [Iqr_ref] -> Product2/3
  Product3/1 -> Sum7/1
  Product16/1 -> Product17/1
  Llr+Lm6/1 -> Product9/2
  Product2/1 -> Sum3/2
  [w] -> Product21/1
  Rotor_Id_ref/1 -> Subsystem/1(Rotor_Id_ref)
  Sum6/1 -> Rotor_conv_Vd/1  "Rotor_conv_Vd"

== system Wind_Turbine_test/Wind Farm/Control System/Control System 1/Rotor-side Control System/Electromagnetic Torque Controller  ==
  Stator_Vdq : Inport
  w : Inport  Port=2
  Stator_Idq : Inport  Port=3
  Tem_cmd : Inport  Port=4
  Divide2 : Product  Inputs=*/
  Divide3 : Product  Inputs=**
  Lm/Ls : Constant  Value=Lm/(Lls+Lm)
  Min_flux-inf : Saturate  UpperLimit=inf  LowerLimit=Flux_min
  Saturation : Saturate  UpperLimit=Idref_max  LowerLimit=0
  Stator flux estimator : Subsystem
  Rotor_Id_ref : Outport
  wires:
  Stator_Idq/1 -> Stator flux estimator/2(Stator_Idq), [Stator_Idq]
  Lm/Ls/1 -> Divide3/2
  Stator flux estimator/1(Mag_Flux) -> Min_flux-inf/1
  Divide2/1 -> Saturation/1
  w/1 -> Stator flux estimator/3(w_pu), [w]
  Min_flux-inf/1 -> Divide3/1
  Saturation/1 -> Rotor_Id_ref/1
  Stator_Vdq/1 -> [Stator_Vdq], Stator flux estimator/1(Stator_Vdq)
  Divide3/1 -> Divide2/2
  Tem_cmd/1 -> Divide2/1

== system Wind_Turbine_test/Wind Farm/Control System/Control System 1/Rotor-side Control System/Iqr, ref_limit ==
  Rotor_Id_ref : Inport
  Constant1 : Constant
  Constant4 : Constant
  Demux4 : Demux  Outputs=2
      settings: DisplayOption=none
  Discrete-Time Integrator2 : DiscreteIntegrator  gainval=10  SampleTime=Ts  LimitOutput=on  UpperSaturationLimit=1  LowerSaturationLimit=0  ICPrevOutput=DiscIntNeverNeededParam  ICPrevScaledInput=DiscIntNeverNeededParam
  Divide1 : Product  Inputs=**
  Irotor_max^2 : Constant
  Math Function : Math  Operator=square  SignedPower=on
  Math Function1 : Math  Operator=sqrt  SignedPower=on
  Math Function2 : Math  Operator=square  SignedPower=on
  Math Function3 : Math  Operator=square  SignedPower=on
  Math Function4 : Math  Operator=sqrt  SignedPower=on
  Sum1 : Sum  Inputs=|-+  InputSameDT=on  SaturateOnIntegerOverflow=on  OutDataTypeStr=Inherit: Same as first input
  Sum10 : Sum  Inputs=|++  InputSameDT=on  SaturateOnIntegerOverflow=on  OutDataTypeStr=Inherit: Same as first input
  Sum11 : Sum  Inputs=|+-  InputSameDT=on  SaturateOnIntegerOverflow=on  OutDataTypeStr=Inherit: Same as first input
  Sum12 : Sum  Inputs=|+-  InputSameDT=on  SaturateOnIntegerOverflow=on  OutDataTypeStr=Inherit: Same as first input
  t=Iq_ref_limit_time_constants : powerlib_extras/Discrete  Control Blocks/Discrete 1st-Order Filter  FilterType=Lowpass  Tc=Iqref_Tc  Ts=Ts  Initialize=on  Vac_Init=[0 0 0]  Vdc_Init=Grid_conv_Imax  PlotResponse=off  param1=[1 500 0.1]
  Iqrlim : Outport
  wires:
  Discrete-Time Integrator2/1 -> Sum12/2
  Sum12/1 -> Divide1/2
  Demux4/2 -> Math Function3/1
  Math Function3/1 -> Sum10/2
  Math Function2/1 -> Sum10/1
  Math Function1/1 -> t=Iq_ref_limit_time_constants/1
  t=Iq_ref_limit_time_constants/1 -> Divide1/1
  Demux4/1 -> Math Function2/1
  Constant1/1 -> Sum11/2
  Constant4/1 -> Sum12/1
  Sum11/1 -> Discrete-Time Integrator2/1
  Math Function/1 -> Sum1/1
  [Stator_Idq] -> Demux4/1
  Sum10/1 -> Math Function4/1
  Irotor_max^2/1 -> Sum1/2
  Rotor_Id_ref/1 -> Math Function/1
  Sum1/1 -> Math Function1/1
  Divide1/1 -> Iqrlim/1  "Iqrlim"
  Math Function4/1 -> Sum11/1

== system Wind_Turbine_test/Wind Farm/Control System/Control System 1/Rotor-side Control System/Modulation Index & Phase ==
  note: m = Vnom_r * 2*sqrt(2/3) / Vdc
  note: Required value for modulation index "m" to obtain 1 pu generated voltage by the converter:
  note: Where Vnom_r = RMS ph-ph nominal voltage
  x : Inport
  y : Inport  Port=2
  Vdc : Inport  Port=3
  0-Mod_index_max_rotor : Saturate  UpperLimit=Rotor_Modindex_Upper  LowerLimit=0
  Avoid division by zero : Saturate  UpperLimit=inf  LowerLimit=1e-6
  Cartesian to Polar : simulink_extras/Transformations/Cartesian to Polar
  K : Constant  Value=Wind_Rotor_V_nom*2*sqrt(2/3)
  Polar to Cartesian : simulink_extras/Transformations/Polar to Cartesian
  Product7 : Product  Inputs=**/  InputSameDT=on  SaturateOnIntegerOverflow=on  OutDataTypeStr=Inherit: Same as first input
  x1 : Outport
  y1 : Outport  Port=2
  wires:
  Vdc/1 -> Avoid division by zero/1
  Product7/1 -> 0-Mod_index_max_rotor/1  "m"
  Polar to Cartesian/1 -> x1/1
  Cartesian to Polar/1 -> Product7/1
  Cartesian to Polar/2 -> Polar to Cartesian/2
  K/1 -> Product7/2
  0-Mod_index_max_rotor/1 -> Polar to Cartesian/1
  Avoid division by zero/1 -> Product7/3
  Polar to Cartesian/2 -> y1/1
  x/1 -> Cartesian to Polar/1
  y/1 -> Cartesian to Polar/2

== system Wind_Turbine_test/Wind Farm/Control System/Control System 1/Rotor-side Control System/Rotor Control Voltage Converter ==
  x1 : Inport
  y1 : Inport  Port=2
  Angle : Inport  Port=3
  Mux4 : Mux  Inputs=3
  Mux5 : Mux  Inputs=2
  Trigonometric Function2 : Trigonometry
  Trigonometric Function3 : Trigonometry  Operator=cos
  V0 : Constant  Value=0
  dq0_to_abc Transformation : powerlib_extras/Measurements/dq0_to_abc Transformation
  Uctrl_rotor_conv : Outport  VectorParamsAs1DForOutWhenUnconnected=off
  wires:
  Mux5/1 -> dq0_to_abc Transformation/2
  Trigonometric Function2/1 -> Mux5/1
  Mux4/1 -> dq0_to_abc Transformation/1  "Vdq0"
  Trigonometric Function3/1 -> Mux5/2
  Angle/1 -> Trigonometric Function3/1, Trigonometric Function2/1
  dq0_to_abc Transformation/1 -> Uctrl_rotor_conv/1
  V0/1 -> Mux4/3
  x1/1 -> Mux4/1
  y1/1 -> Mux4/2

== system Wind_Turbine_test/Wind Farm/Control System/Control System 1/Rotor-side Control System/Var Regulator ==
  Qref : Inport
  Meas_Q : Inport  Port=2
  Meas_V : Inport  Port=3
  Discrete-Time Integrator1 : DiscreteIntegrator  gainval=Ki_Var  InitialConditionSource=external  InitialCondition=1  SampleTime=Ts  LimitOutput=on  UpperSaturationLimit=Var_reg_max  LowerSaturationLimit=Var_reg_min  ICPrevOutput=DiscIntNeverNeededParam  ICPrevScaledInput=DiscIntNeverNeededParam
  Sum : Sum  Inputs=|-+  InputSameDT=on  SaturateOnIntegerOverflow=on  OutDataTypeStr=Inherit: Same as first input
  Sum2 : Sum  Inputs=|+-  InputSameDT=on  SaturateOnIntegerOverflow=on  OutDataTypeStr=Inherit: Same as first input
  Unit Delay1 : UnitDelay  InitialCondition=1  SampleTime=Ts  HasFrameUpgradeWarning=on
  Out1 : Outport
  wires:
  Discrete-Time Integrator1/1 -> Sum/1  "Vref"
  Meas_V/1 -> Unit Delay1/1, Sum/2
  Sum2/1 -> Discrete-Time Integrator1/1
  Unit Delay1/1 -> Discrete-Time Integrator1/2
  Qref/1 -> Sum2/1
  Meas_Q/1 -> Sum2/2
  Sum/1 -> Out1/1

== system Wind_Turbine_test/Wind Farm/Control System/Control System 1/Rotor-side Control System/Voltage Regulator ==
  Max : Inport
  Min : Inport  Port=2
  In : Inport  Port=3
  Constant2 : Constant  Value=0
  Constant3 : Constant  Value=Ki_Vreg
  Data Type Conversion2 : DataTypeConversion  OutDataTypeStr=boolean  SaturateOnIntegerOverflow=off  RndMeth=Floor
  Gain : Gain  Gain=-1  SaturateOnIntegerOverflow=on  OutDataTypeStr=Inherit: Same as input  ParamDataTypeStr=Inherit: Same as input
  INT : Subsystem  mask(Integrator  With  External  Dynamic  Limits (Discrete)){}
      mask Display: disp('Discrete-Time\n(Trapezoidal)\nIntegrator\n ')
  Iqr_ref : Outport
  wires:
  Min/1 -> Gain/1
  Data Type Conversion2/1 -> INT/6(Reset), INT/5(Hold)
  Constant3/1 -> INT/4(Ki)
  Constant2/1 -> INT/7(Reset Value), Data Type Conversion2/1
  Max/1 -> INT/1(Max)
  Gain/1 -> INT/2(Min)
  INT/1(Out) -> Iqr_ref/1
  In/1 -> INT/3(In)

== system Wind_Turbine_test/Wind Farm/Control System/Control System 1/Speed & Pitch Control System/Discrete PI Controller ==
  note: Discrete PID Controller
  note: Pierre Giroux, Gilbert Sybille
      | Power System Simulation Laboratory
      | IREQ, Hydro-Quebc
  Error : Inport
  Discrete-Time Integrator : DiscreteIntegrator  InitialCondition=Init  SampleTime=Ts  LimitOutput=on  UpperSaturationLimit=UpperLimit  LowerSaturationLimit=LowerLimit  ICPrevOutput=DiscIntNeverNeededParam  ICPrevScaledInput=DiscIntNeverNeededParam
  Product1 : Product  RndMeth=Zero
  Product2 : Product  RndMeth=Zero
  Saturation2 : Saturate  UpperLimit=UpperLimit  LowerLimit=LowerLimit
  Step_Ki_speed : Step  Time=999  Before=Ki  After=Ki  SampleTime=Ts
  Step_Kp_speed : Step  Time=999  Before=Kp  After=Kp  SampleTime=Ts
  Sum6 : Sum  InputSameDT=on  SaturateOnIntegerOverflow=on  OutDataTypeStr=Inherit: Same as first input
  Out : Outport  InitialOutput=0  VectorParamsAs1DForOutWhenUnconnected=off
  wires:
  Saturation2/1 -> Out/1
  Discrete-Time Integrator/1 -> Sum6/2
  Product1/1 -> Sum6/1
  Product2/1 -> Discrete-Time Integrator/1
  Sum6/1 -> Saturation2/1
  Error/1 -> Product1/2, Product2/1
  Step_Kp_speed/1 -> Product1/1
  Step_Ki_speed/1 -> Product2/2

== system Wind_Turbine_test/Wind Farm/Control System/Control System 2/Grid-side Control System/Current Regulator ==
  Stator_Vdq : Inport
  In2 : Inport  Port=2
  Grid_conv_Idq : Inport  Port=3
  w : Inport  Port=4
  Constant1 : Constant  Value=L_pu
  Constant2 : Constant  Value=L_pu
  Constant3 : Constant  Value=R_pu
  Constant4 : Constant  Value=R_pu
  Demux{,1..3} (4 alike) : Demux  Outputs=2
      settings: DisplayOption=none
  Discrete PI Controller1 : powerlib_extras/Discrete  Control Blocks/Discrete PI Controller  Kp=Grid_Ireg_Kp  Ki=Grid_Ireg_Ki  Par_Limits=[1.0 -1.0] *Grid_Ireg_lim  Init=0  Ts=Ts
  Mux2 : Mux  Inputs=2
  Product : Product  Inputs=3  InputSameDT=on  SaturateOnIntegerOverflow=on  OutDataTypeStr=Inherit: Same as first input
  Product1 : Product  Inputs=3  InputSameDT=on  SaturateOnIntegerOverflow=on  OutDataTypeStr=Inherit: Same as first input
  Product2 : Product  InputSameDT=on  SaturateOnIntegerOverflow=on  OutDataTypeStr=Inherit: Same as first input
  Product3 : Product  InputSameDT=on  SaturateOnIntegerOverflow=on  OutDataTypeStr=Inherit: Same as first input
  Sum1 : Sum  Inputs=+-  InputSameDT=on  SaturateOnIntegerOverflow=on  OutDataTypeStr=Inherit: Same as first input
  Sum2 : Sum  Inputs=-+|  InputSameDT=on  SaturateOnIntegerOverflow=on  OutDataTypeStr=Inherit: Same as first input
  Sum3 : Sum  Inputs=||++-  InputSameDT=on  SaturateOnIntegerOverflow=on  OutDataTypeStr=Inherit: Same as first input
  Sum4 : Sum  Inputs=|+-  InputSameDT=on  SaturateOnIntegerOverflow=on  OutDataTypeStr=Inherit: Same as first input
  Sum5 : Sum  Inputs=|--+  InputSameDT=on  SaturateOnIntegerOverflow=on  OutDataTypeStr=Inherit: Same as first input
  Sum6 : Sum  Inputs=|-+  InputSameDT=on  SaturateOnIntegerOverflow=on  OutDataTypeStr=Inherit: Same as first input
  Grid_conv_Vd : Outport
  Grid_conv_Vq : Outport  Port=2
  wires:
  Product1/1 -> Sum5/2
  Product2/1 -> Sum3/3
  Product3/1 -> Sum5/1
  [id_ref] -> Product2/2
  Sum1/1 -> Grid_conv_Vd/1  "Grid_conv_Vd"
  Demux1/2 -> [iq_ref], Sum2/2  "Iq_ref"
  Demux/1 -> Sum4/2  "Id"
  [w] -> Product/2
  Demux2/2 -> Sum5/3  "Vq"
  [iq_ref] -> Product/3
  Sum4/1 -> Mux2/1
  Constant4/1 -> Product3/2
  Stator_Vdq/1 -> Demux2/1
  Constant2/1 -> Product1/2
  Constant3/1 -> Product2/1
  Grid_conv_Idq/1 -> Demux/1
  Product/1 -> Sum3/2
  Discrete PI Controller1/1 -> Demux3/1
  Sum2/1 -> Mux2/2
  Sum6/1 -> Grid_conv_Vq/1  "Grid_conv_Vq"
  w/1 -> [w]
  [id_ref] -> Product1/1
  Sum5/1 -> Sum6/2
  [iq_ref] -> Product3/1
  Sum3/1 -> Sum1/1
  Mux2/1 -> Discrete PI Controller1/1
  Demux2/1 -> Sum3/1  "Vd"
  Demux1/1 -> Sum4/1, [id_ref]  "Id_ref"
  Demux3/1 -> Sum1/2  "vd'"
  Constant1/1 -> Product/1
  Demux/2 -> Sum2/1  "Iq"
  Demux3/2 -> Sum6/1  "vq'"
  [w] -> Product1/3
  In2/1 -> Demux1/1
